simulink model "kalman_oscillator_2021_04_22"  (R2020a)
settings: Solver=ode23tb  StartTime=0.0  StopTime=simlength  MaxStep=Ts
undefined symbols (not defined in the file): Afd, Bfd, Cf, ki, kp, magnitude, qkalman, Rkalman, Tc, Ts, w
libraries: simulink x1, cstblocks x1
settings Model: SimulationMode=accelerator  Creator=dbagn  LastModifiedBy=dabagnara
settings SolverCC: SolverResetMethod=Robust
settings DataIOCC: ReturnWorkspaceOutputs=off

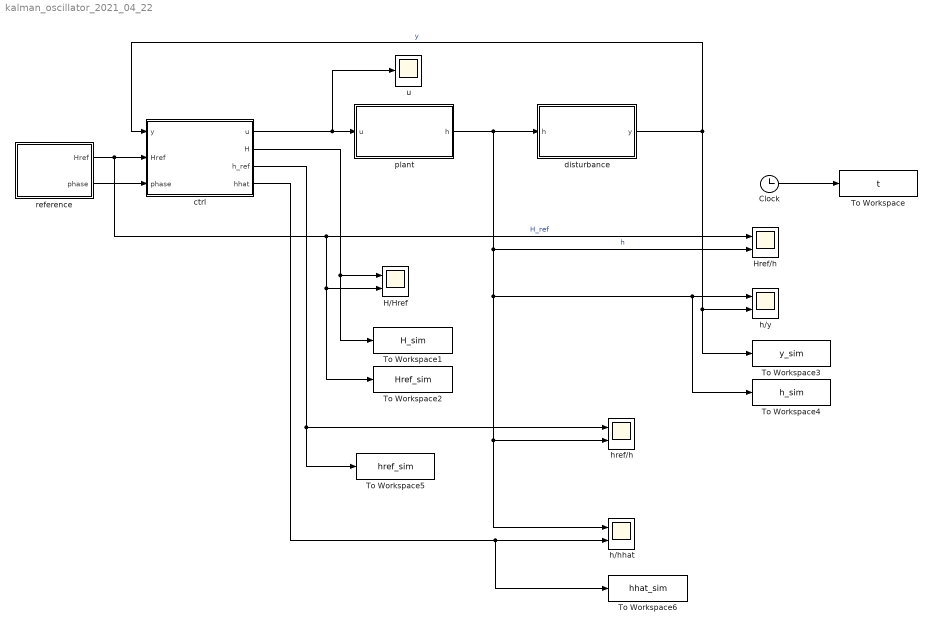
== system kalman_oscillator_2021_04_22 ==
  Clock : Clock
  H/Href : Scope  NumInputPorts=2
  Href/h : Scope  NumInputPorts=2
  To Workspace : ToWorkspace  VariableName=t  SampleTime=Tc
      settings: MaxDataPoints=Nc
  To Workspace1 : ToWorkspace  VariableName=H_sim  SampleTime=Tc
      settings: MaxDataPoints=Nc
  To Workspace2 : ToWorkspace  VariableName=Href_sim  SampleTime=Tc
      settings: MaxDataPoints=Nc
  To Workspace3 : ToWorkspace  VariableName=y_sim  SampleTime=Tc
      settings: MaxDataPoints=Nc
  To Workspace4 : ToWorkspace  VariableName=h_sim  SampleTime=Tc
      settings: MaxDataPoints=Nc
  To Workspace5 : ToWorkspace  VariableName=href_sim  SampleTime=Tc
      settings: MaxDataPoints=Nc
  To Workspace6 : ToWorkspace  VariableName=hhat_sim  SampleTime=Tc
      settings: MaxDataPoints=Nc
  ctrl : Subsystem
  disturbance : Subsystem
  h/hhat : Scope  NumInputPorts=2
  h/y : Scope  NumInputPorts=2
  href/h : Scope  NumInputPorts=2
  plant : Subsystem
  reference : Subsystem
  u : Scope
  wires:
  reference/1(Href) -> To Workspace2/1, H/Href/2, Href/h/1, ctrl/2(Href)  "H_ref"
  ctrl/1(u) -> u/1, plant/1(u)
  plant/1(h) -> Href/h/2, To Workspace4/1, h/y/1, href/h/2, h/hhat/1, disturbance/1(h)  "h"
  disturbance/1(y) -> To Workspace3/1, h/y/2, ctrl/1(y)  "y"
  reference/2(phase) -> ctrl/3(phase)
  ctrl/2(H) -> To Workspace1/1, H/Href/1
  Clock/1 -> To Workspace/1
  ctrl/3(h_ref) -> To Workspace5/1, href/h/1
  ctrl/4(hhat) -> To Workspace6/1, h/hhat/2

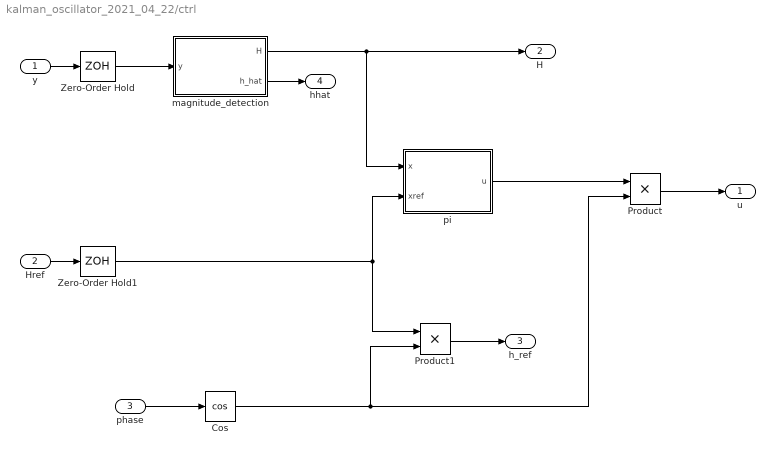
== system kalman_oscillator_2021_04_22/ctrl ==
  y : Inport
  Href : Inport  Port=2
  phase : Inport  Port=3
  Cos : Trigonometry  Operator=cos
  Product : Product
  Product1 : Product
  Zero-Order Hold : ZeroOrderHold  SampleTime=Ts
  Zero-Order Hold1 : ZeroOrderHold  SampleTime=Ts
  magnitude_detection : Subsystem
  pi : Subsystem  mask{kp=kp, ki=ki, ts=Ts, sat_pos=inf, sat_neg=-inf}
  u : Outport  VectorParamsAs1DForOutWhenUnconnected=off
  H : Outport  Port=2  VectorParamsAs1DForOutWhenUnconnected=off
  h_ref : Outport  Port=3  VectorParamsAs1DForOutWhenUnconnected=off
  hhat : Outport  Port=4  VectorParamsAs1DForOutWhenUnconnected=off
  wires:
  Href/1 -> Zero-Order Hold1/1
  y/1 -> Zero-Order Hold/1
  magnitude_detection/1(H) -> pi/1(x), H/1
  Zero-Order Hold/1 -> magnitude_detection/1(y)
  Zero-Order Hold1/1 -> pi/2(xref), Product1/1
  phase/1 -> Cos/1
  Cos/1 -> Product/2, Product1/2
  Product/1 -> u/1
  Product1/1 -> h_ref/1
  magnitude_detection/2(h_hat) -> hhat/1
  pi/1(u) -> Product/1

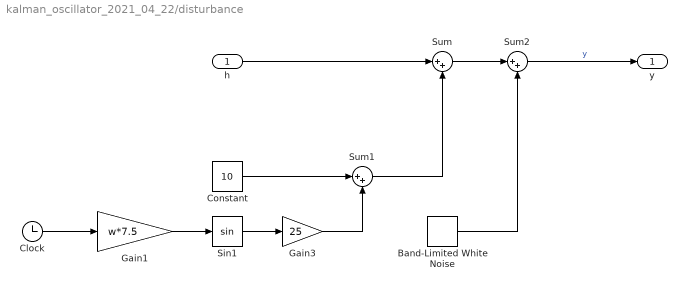
== system kalman_oscillator_2021_04_22/disturbance ==
  h : Inport
  Band-Limited White Noise : simulink/Sources/Band-Limited White Noise  Cov=Tc  Ts=Tc  seed=[23341]
  Clock : Clock
  Constant : Constant  Value=10
  Gain1 : Gain  Gain=w*7.5
  Gain3 : Gain  Gain=25
  Sin1 : Trigonometry
  Sum : Sum  Inputs=|++
  Sum1 : Sum  Inputs=|++
  Sum2 : Sum  Inputs=|++
  y : Outport
  wires:
  Gain3/1 -> Sum1/2
  Band-Limited White Noise/1 -> Sum2/2
  Sin1/1 -> Gain3/1
  Clock/1 -> Gain1/1
  Sum/1 -> Sum2/1
  Constant/1 -> Sum1/1
  Sum2/1 -> y/1  "y"
  Sum1/1 -> Sum/2
  Gain1/1 -> Sin1/1
  h/1 -> Sum/1

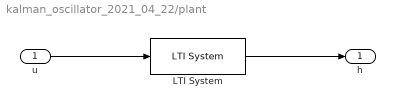
== system kalman_oscillator_2021_04_22/plant ==
  u : Inport
  LTI System : cstblocks/LTI System  sys=plant  IC=[]
  h : Outport  VectorParamsAs1DForOutWhenUnconnected=off
  wires:
  LTI System/1 -> h/1
  u/1 -> LTI System/1

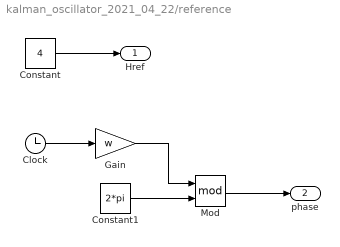
== system kalman_oscillator_2021_04_22/reference ==
  Clock : Clock
  Constant : Constant  Value=4
  Constant1 : Constant  Value=2*pi
  Gain : Gain  Gain=w
  Mod : Math  Operator=mod  SaturateOnIntegerOverflow=on
  Href : Outport
  phase : Outport  Port=2
  wires:
  Clock/1 -> Gain/1
  Constant/1 -> Href/1
  Constant1/1 -> Mod/2
  Gain/1 -> Mod/1
  Mod/1 -> phase/1

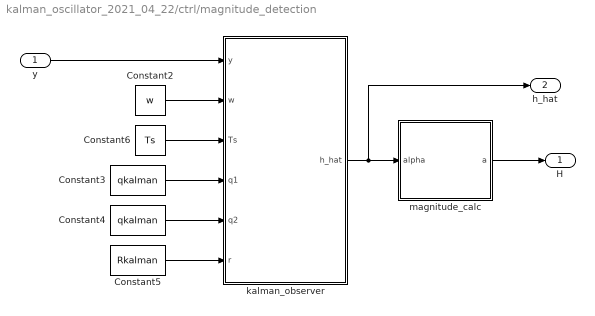
== system kalman_oscillator_2021_04_22/ctrl/magnitude_detection ==
  y : Inport
  Constant2 : Constant  Value=w
  Constant3 : Constant  Value=qkalman
  Constant4 : Constant  Value=qkalman
  Constant5 : Constant  Value=Rkalman
  Constant6 : Constant  Value=Ts
  kalman_observer : MATLAB Function  TreatAsAtomicUnit=on  SystemSampleTime=Ts
  magnitude_calc : Subsystem
  H : Outport
  h_hat : Outport  Port=2
  wires:
  Constant2/1 -> kalman_observer/2(w)
  y/1 -> kalman_observer/1(y)
  Constant6/1 -> kalman_observer/3(Ts)
  Constant5/1 -> kalman_observer/6(r)
  magnitude_calc/1(a) -> H/1
  Constant3/1 -> kalman_observer/4(q1)
  Constant4/1 -> kalman_observer/5(q2)
  kalman_observer/1(h_hat) -> h_hat/1, magnitude_calc/1(alpha)

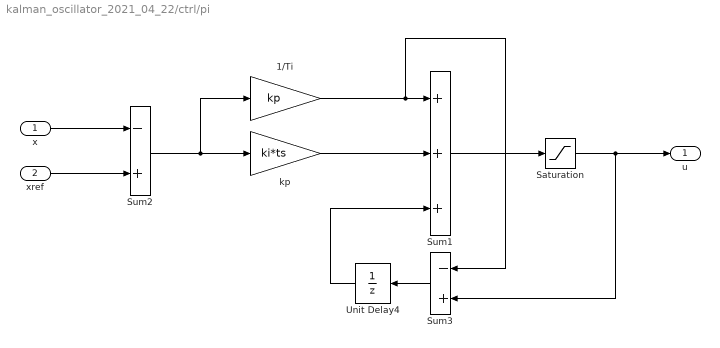
== system kalman_oscillator_2021_04_22/ctrl/pi ==
  x : Inport
  xref : Inport  Port=2
  1/Ti : Gain  Gain=kp  SaturateOnIntegerOverflow=on  OutDataTypeStr=Inherit: Same as input  ParamDataTypeStr=Inherit: Same as input
  Saturation : Saturate  UpperLimit=sat_pos  LowerLimit=sat_neg
  Sum1 : Sum  Inputs=+++  SaturateOnIntegerOverflow=on
  Sum2 : Sum  Inputs=-+  SaturateOnIntegerOverflow=on
  Sum3 : Sum  Inputs=-+  SaturateOnIntegerOverflow=on
  Unit Delay4 : UnitDelay  SampleTime=ts  HasFrameUpgradeWarning=on
  kp : Gain  Gain=ki*ts  SaturateOnIntegerOverflow=on  OutDataTypeStr=Inherit: Same as input  ParamDataTypeStr=Inherit: Same as input
  u : Outport
  wires:
  xref/1 -> Sum2/2
  kp/1 -> Sum1/2
  Sum2/1 -> kp/1, 1/Ti/1
  1/Ti/1 -> Sum1/1, Sum3/1
  Sum3/1 -> Unit Delay4/1
  x/1 -> Sum2/1
  Sum1/1 -> Saturation/1
  Unit Delay4/1 -> Sum1/3
  Saturation/1 -> u/1, Sum3/2

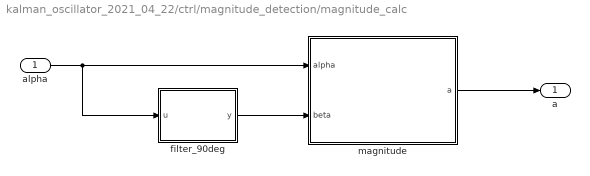
== system kalman_oscillator_2021_04_22/ctrl/magnitude_detection/magnitude_calc ==
  alpha : Inport
  filter_90deg : Subsystem
  magnitude : Subsystem
  a : Outport
  wires:
  magnitude/1(a) -> a/1
  alpha/1 -> filter_90deg/1(u), magnitude/1(alpha)
  filter_90deg/1(y) -> magnitude/2(beta)

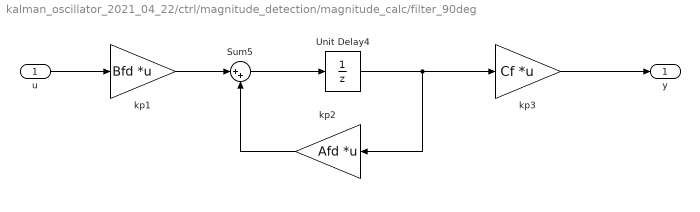
== system kalman_oscillator_2021_04_22/ctrl/magnitude_detection/magnitude_calc/filter_90deg ==
  u : Inport
  Sum5 : Sum  Inputs=|++
  Unit Delay4 : UnitDelay  SampleTime=Ts  HasFrameUpgradeWarning=on
  kp1 : Gain  Gain=Bfd  Multiplication=Matrix(K*u)  SaturateOnIntegerOverflow=on  OutDataTypeStr=Inherit: Same as input  ParamDataTypeStr=Inherit: Same as input
  kp2 : Gain  Gain=Afd  Multiplication=Matrix(K*u)  SaturateOnIntegerOverflow=on  OutDataTypeStr=Inherit: Same as input  ParamDataTypeStr=Inherit: Same as input
  kp3 : Gain  Gain=Cf  Multiplication=Matrix(K*u)  SaturateOnIntegerOverflow=on  OutDataTypeStr=Inherit: Same as input  ParamDataTypeStr=Inherit: Same as input
  y : Outport
  wires:
  Unit Delay4/1 -> kp2/1, kp3/1
  Sum5/1 -> Unit Delay4/1
  kp3/1 -> y/1
  kp2/1 -> Sum5/2
  kp1/1 -> Sum5/1
  u/1 -> kp1/1

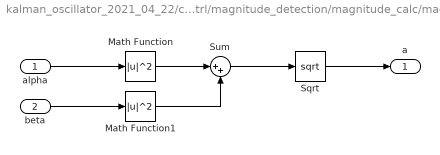
== system kalman_oscillator_2021_04_22/ctrl/magnitude_detection/magnitude_calc/magnitude ==
  alpha : Inport
  beta : Inport  Port=2
  Math Function : Math  Operator=magnitude^2  SaturateOnIntegerOverflow=on
  Math Function1 : Math  Operator=magnitude^2  SaturateOnIntegerOverflow=on
  Sqrt : Sqrt  SaturateOnIntegerOverflow=on
  Sum : Sum  Inputs=|++
  a : Outport
  wires:
  alpha/1 -> Math Function/1
  beta/1 -> Math Function1/1
  Math Function/1 -> Sum/1
  Math Function1/1 -> Sum/2
  Sum/1 -> Sqrt/1
  Sqrt/1 -> a/1

== matlab function kalman_oscillator_2021_04_22/ctrl/magnitude_detection/kalman_observer ==
  data: y input; h_hat output; w input; Ts input; q1 input; q2 input; r input
function h_hat   = KFO(y,w,Ts,q1,q2,r)

    persistent   x1_po x2_po p11_po p12_po p21_po p22_po

    if isempty(x1_po)
        x1_po = 0;
        x2_po = 0;
        p11_po = 0;
        p12_po = 0;
        p21_po = 0;
        p22_po = 0;        
    end
    
    a11 = cos(w*Ts);
    a12 = sin(w*Ts);
    a21 = -sin(w*Ts);
    a22 = cos(w*Ts);
   
    
    
    x1_pr = a11*x1_po + a12*x2_po;
    x2_pr = a21*x1_po + a22*x2_po;
    
    p11_pr = q1 + a11*(a11*p11_po+a12*p21_po) + a12*(a11*p12_po+a12*p22_po);
    p12_pr = a21*(a11*p11_po+a12*p21_po) + a22*(a11*p12_po+a12*p22_po);
    p21_pr = a11*(a21*p11_po+a22*p21_po) + a12*(a21*p12_po+a22*p22_po);
    p22_pr = q2 + a21*(a21*p11_po+a22*p21_po) + a22*(a21*p12_po+a22*p22_po);
    
    l1 = p11_pr/(p11_pr + r);
    l2 = p21_pr/(p11_pr + r);
    
    x1_po = x1_pr + l1*(y-x1_pr);
    x2_po = x2_pr + l2*(y-x1_pr);
    
    p11_po = (1-l1)*p11_pr;
    p12_po = (1-l1)*p12_pr;
    p21_po = p21_pr-l2*p11_pr;
    p22_po = p22_pr-l2*p12_pr;
    
    
    
    h_hat = x1_pr;
end
